simulink model "req4"  (R2019a)
settings: Solver=FixedStepAuto  StartTime=0.0  StopTime=100  RelTol=1e-3
settings Model: Creator=e40014285  LastModifiedBy=e40014285
settings ConfigComp: CovScope=ReferencedModels  CovIncludeTopModel=off

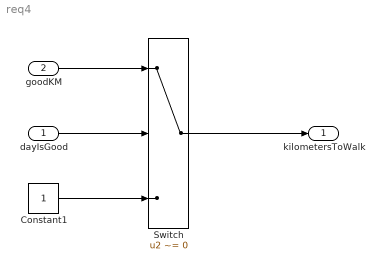
== system req4 ==
  dayIsGood : Inport  OutDataTypeStr=double
  goodKM : Inport  Port=2  OutDataTypeStr=double
  Constant1 : Constant
  Switch : Switch  Criteria=u2 ~= 0
  kilometersToWalk : Outport
  wires:
  dayIsGood/1 -> Switch/2
  Switch/1 -> kilometersToWalk/1
  goodKM/1 -> Switch/1
  Constant1/1 -> Switch/3
